simulink model "BicycleTestModel"  (R2021b)
settings: Solver=VariableStepAuto  StartTime=0.0  StopTime=250  RelTol=1e-3
libraries: simulink x2, slpidlib x1
settings Model: Creator=jpchi  LastModifiedBy=jpchi
settings SolverCC: AlgebraicLoopSolver=TrustRegion
settings DebuggingCC: SFMachineParentedDataDiag=warning

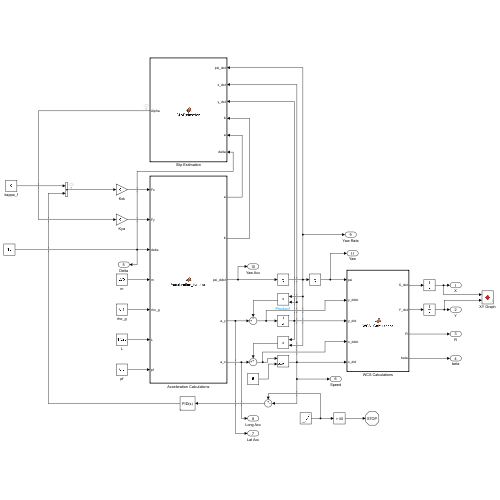
[thumbnail: Simulink's stored preview of the top-level diagram]
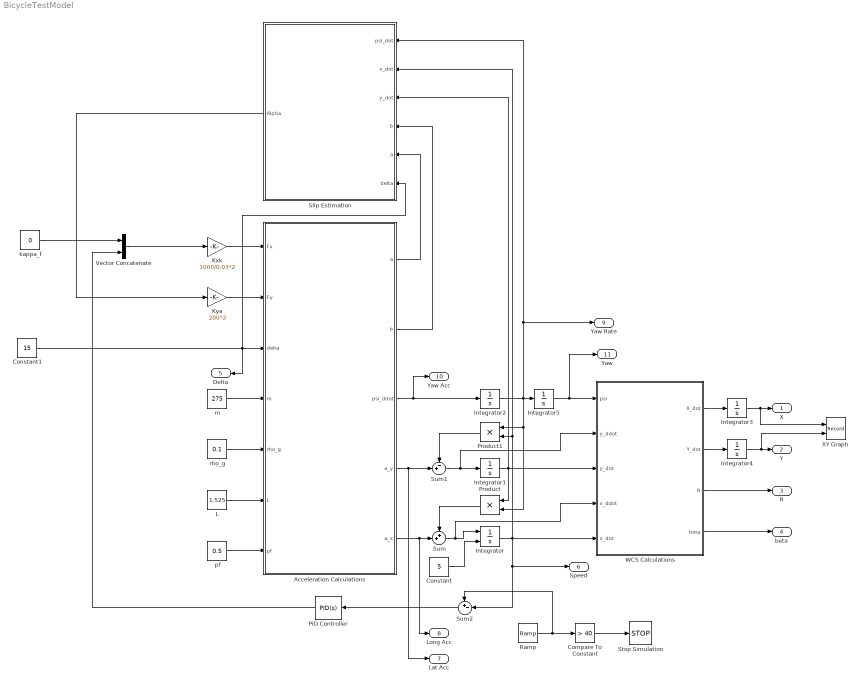
== system BicycleTestModel ==
  Acceleration Calculations : MATLAB Function  TreatAsAtomicUnit=on
  Compare To Constant : simulink/Logic and Bit Operations/Compare To Constant  relop=>  const=40  OutDataTypeStr=boolean
  Constant : Constant  Value=5
  Constant1 : Constant  Value=15
  Integrator : Integrator  InitialConditionSource=external  InitialCondition=15
  Integrator{1..5} (5 alike) : Integrator
  Kxk : Gain  Gain=1000/0.03*2
  Kya : Gain  Gain=200*2
  L : Constant  Value=1.525
  PID Controller : slpidlib/PID Controller  Controller=PID  Form=Parallel  TimeDomain=Continuous-time  UseExternalTs=off  SampleTime=-1  IntegratorMethod=Forward Euler  FilterMethod=Forward Euler  ControllerParametersSource=internal  P=0.0412468421192802  I=0.00360891443153185  D=3.60919075314681e-05  UseFilter=on  N=1142.8279760416  TunerSelectOption=Transfer Function Based (PID Tuner App)  InitialConditionSource=internal  InitialConditionForIntegrator=0  InitialConditionForFilter=0  DifferentiatorICPrevScaledInput=0  ExternalReset=none  TrackingMode=off  Kt=1  LimitOutput=off  SatLimitsSource=internal  UpperSaturationLimit=inf  LowerSaturationLimit=-inf  LinearizeAsGain=on  AntiWindupMode=none  Kb=1  POutMin=[]  POutMax=[]  IOutMin=[]  IOutMax=[]  DOutMin=[]  DOutMax=[]  NOutMin=[]  NOutMax=[]  SumOutMin=[]  SumOutMax=[]  SaturationOutMin=[]  SaturationOutMax=[]  PParamMin=[]  PParamMax=[]  IParamMin=[]  IParamMax=[]  DParamMin=[]  DParamMax=[]  NParamMin=[]  NParamMax=[]  KbParamMin=[]  KbParamMax=[]  KtParamMin=[]  KtParamMax=[]  KbOutMin=[]  KbOutMax=[]  KtOutMin=[]  KtOutMax=[]  IntegratorOutMin=[]  IntegratorOutMax=[]  FilterOutMin=[]  FilterOutMax=[]  SumI1OutMin=[]  SumI1OutMax=[]  SumI2OutMin=[]  SumI2OutMax=[]  SumI3OutMin=[]  SumI3OutMax=[]  SumI4OutMin=[]  SumI4OutMax=[]  SumDOutMin=[]  SumDOutMax=[]  DifferentiatorOutMin=[]  DifferentiatorOutMax=[]  FilterDiffOutCoefMin=[]  FilterDiffOutCoefMax=[]  ReciprocalOutMin=[]  ReciprocalOutMax=[]  SumDenOutMin=[]  SumDenOutMax=[]  SumNumOutMin=[]  SumNumOutMax=[]  DivideOutMin=[]  DivideOutMax=[]  UdiffTsProdOutMin=[]  UdiffTsProdOutMax=[]  NTsProdOutMin=[]  NTsProdOutMax=[]  UintegralTsProdOutMin=[]  UintegralTsProdOutMax=[]  UngainTsProdOutMin=[]  UngainTsProdOutMax=[]  IntegratorContinuousStateAttributes=''  IntegratorStateMustResolveToSignalObject=off  IntegratorRTWStateStorageClass=Auto  FilterContinuousStateAttributes=''  FilterStateMustResolveToSignalObject=off  FilterRTWStateStorageClass=Auto  ParallelPVariant=InternalParameters  IdealPVariant=Disabled  IVariant=InternalParameters  DVariant=InternalParameters  IntegratorVariant=Continuous  SatVariant=Disabled  AWVariant=Passthrough  PCopyVariant=Disabled  TRVariant=Disabled  FdbkBlocksVariant=Forward  IdealPFdbkVariant=Disabled  SatFdbkVariant=Disabled  DerivativeFilterVariant=ContFilter  NVariant=InternalParameters  NCopyVariant=Disabled  FilterICVariant=InternalICsFilter  IntegratorICVariant=InternalICs  ExternalResetVariant=Disabled  TRSumVariant=Passthrough  SumFdbkVariant=Disabled  SumVariant=Sum_PID  TsampFilterVariant=InternalTs  TsampNgainVariant=Passthrough  TsampIntegralVariant=Passthrough  ExternalSaturationOutDataTypeStr=Inherit: Same as second input
  Product : Product
  Product1 : Product
  Ramp : simulink/Sources/Ramp  slope=0.05  start=0  InitialOutput=5
  Slip Estimation : MATLAB Function  TreatAsAtomicUnit=on
  Stop Simulation : Stop
  Sum : Sum  Inputs=++|
  Sum1 : Sum  Inputs=-+|
  Sum2 : Sum  Inputs=+-|
  Vector Concatenate : Concatenate
  WCS Calculations : MATLAB Function  TreatAsAtomicUnit=on
  XY Graph : Record  FileSettingsInternal="{\"entries\":[{\"content\":{\"excelSettings\":{\"content\":{},\"type\":\"Streamout.ExcelSettings\"}},\"type\":\"Streamout.FileSettingStorage\",\"uuid\":\"7ebcfab8-f0b6-44cf-b331-51be0f9892d2\"}],\"packageUris\":[\"http://schema.mathworks.com/mf0/streamout_blocks/R2020a\"],\"version\":\"1.0\"}"  Layout=[1 1]  SignalsInternal="{\"entries\":[{\"content\":{\"signals\":[{\"content\":{\"blockPath\":[\"BicycleTestModel/XY Graph\"],\"channel\":[],\"dimensions\":[1],\"domain\":\"BicycleTestModel/XY Graph\",\"lineColor\":\"#a2142f\",\"plots\":[1],\"port\":1,\"sid\":[\"\"],\"signalID\":78,\"signalName\":\"Integrator3\"},\"type\":\"RecordBlkView.Signal\",\"uuid\":\"63fa4d83-aa3b-45f8-8409-7f1995dd79e0\"},{\"content\":{\"blockPath\":[\"BicycleTestModel/XY Graph\"],\"channel\":[],\"dimensions\":[1],\"domain\":\"BicycleTestModel/XY Graph\",\"lineColor\":\"#139fff\",\"plots\":[1],\"port\":2,\"sid\":[\"\"],\"signalID\":82,\"signalName\":\"Integrator4\"},\"type\":\"RecordBlkView.Signal\",\"uuid\":\"d2e667c4-aec6-4e2b-94b9-9e656a73197c\"}]},\"type\":\"RecordBlkView.InputSignals\",\"uuid\":\"f7a6955a-d84c-488f-aee4-1c970144e732\"}],\"packageUris\":[\"http://schema.mathworks.com/mf0/streamout_blocks/R2020a\"],\"version\":\"1.0\"}"  VisualizationBindings="{\"xyplotplugin\":{\"info\":[{\"series\":[{\"bindingParametersList\":[{\"parameter\":\"X-Axis\",\"signalID\":78,\"signalName\":\"Integrator3\"},{\"parameter\":\"Y-Axis\",\"signalID\":82,\"signalName\":\"Integrator4\"}],\"seriesID\":51605}],\"subplotID\":1}]}}"  CompatibilityTag=XY  st=-1
  kappa_f : Constant  Value=0
  m : Constant  Value=275
  pf : Constant  Value=0.5
  rho_g : Constant  Value=0.1
  X : Outport
  Y : Outport  Port=2
  R : Outport  Port=3
  beta : Outport  Port=4
  Delta : Outport  Port=5
  Speed : Outport  Port=6
  Lat Acc : Outport  Port=7
  Long Acc : Outport  Port=8
  Yaw Rate : Outport  Port=9
  Yaw Acc : Outport  Port=10
  Yaw : Outport  Port=11
  wires:
  m/1 -> Acceleration Calculations/4(m)
  rho_g/1 -> Acceleration Calculations/5(rho_g)
  Kxk/1 -> Acceleration Calculations/1(Fx)
  Slip Estimation/1(Alpha) -> Kya/1
  Kya/1 -> Acceleration Calculations/2(Fy)
  Constant1/1 -> Delta/1, Slip Estimation/6(delta), Acceleration Calculations/3(delta)
  Sum/1 -> WCS Calculations/4(x_ddot), Integrator/1
  Sum1/1 -> WCS Calculations/2(y_ddot), Integrator1/1
  Acceleration Calculations/3(psi_ddot) -> Yaw Acc/1, Integrator2/1
  Integrator1/1 -> WCS Calculations/3(y_dot), Slip Estimation/3(y_dot), Product/1
  Integrator2/1 -> Yaw Rate/1, Slip Estimation/1(psi_dot), Product/2, Product1/1, Integrator5/1
  Integrator/1 -> WCS Calculations/5(x_dot), Slip Estimation/2(x_dot), Product1/2, Speed/1, Sum2/2
  L/1 -> Acceleration Calculations/6(L)
  pf/1 -> Acceleration Calculations/7(pf)
  Constant/1 -> Integrator/2
  Acceleration Calculations/5(a_x) -> Long Acc/1, Sum/2
  Product/1 -> Sum/1
  Acceleration Calculations/4(a_y) -> Lat Acc/1, Sum1/2
  Product1/1 -> Sum1/1
  Acceleration Calculations/1(a) -> Slip Estimation/5(a)
  Acceleration Calculations/2(b) -> Slip Estimation/4(b)
  Sum2/1 -> PID Controller/1
  Integrator5/1 -> Yaw/1, WCS Calculations/1(psi)
  WCS Calculations/1(X_dot) -> Integrator3/1
  WCS Calculations/2(Y_dot) -> Integrator4/1
  Integrator3/1 -> XY Graph/1, X/1
  Integrator4/1 -> XY Graph/2, Y/1
  WCS Calculations/3(R) -> R/1
  WCS Calculations/4(beta) -> beta/1
  Vector Concatenate/1 -> Kxk/1
  kappa_f/1 -> Vector Concatenate/1
  PID Controller/1 -> Vector Concatenate/2
  Ramp/1 -> Sum2/1, Compare To Constant/1
  Compare To Constant/1 -> Stop Simulation/1

== matlab function BicycleTestModel/Slip Estimation ==
  data: psi_dot input; x_dot input; Alpha output; y_dot input; b input; a input; delta input
function Alpha = SlipEstimation(psi_dot, x_dot, y_dot, b, a, delta)

Alpha = zeros(1,2);

Alpha(1) = delta - atan2d( y_dot + a*psi_dot, x_dot );
Alpha(2) = -atan2d( y_dot - b.*psi_dot, x_dot );

== matlab function BicycleTestModel/Acceleration Calculations ==
  data: a output; b output; psi_ddot output; a_y output; Fx input size=[1 2]; a_x output; Fy input size=[1 2]; delta input; m input; rho_g input; L input; pf input
function [a, b, psi_ddot, a_y, a_x] = ...
    Acceleration_function(Fx,Fy,delta,m,rho_g,L,pf)
%%% Took out data parameer
%% Parameter
a = L* (1-pf);
b = L*pf;

Izz = m*(rho_g)^2;

%% Longitudinal 
a_x = ( Fx(1)*cosd(delta) - Fy(1)*sind(delta) + Fx(2) ) / m;

%% Lateral
a_y = ( Fy(1)*cosd(delta) + Fx(1)*sind(delta) + Fy(2) ) / m;

%% Yaw
psi_ddot = ( a*( Fy(1)*cosd(delta) + Fx(1)*sind(delta) ) - b*Fy(2) ) / Izz;

end

== matlab function BicycleTestModel/WCS Calculations ==
  data: psi input; y_ddot input; y_dot input; x_ddot input; x_dot input; X_dot output; Y_dot output; R output; beta output
function [X_dot, Y_dot, R, beta] = ...
    WCS_Calculations( psi, y_ddot, y_dot, x_ddot, x_dot )
%% Global Velocity
X_dot = x_dot .* cosd( psi ) - y_dot .* sind( psi );
Y_dot = x_dot .* sind( psi ) + y_dot .* cosd( psi );  
                 
%% Curvature
if abs(x_dot.^2 + y_dot.^2) <= 0.01
    R = 0;
else
    R = ( y_dot.^2 + y_dot.^2 ).^(3/2) ./ ...
        abs( x_ddot.*y_dot - x_dot.*y_ddot );
end

%% Body Slip
beta = atan2d( y_dot, x_dot );
